simulink model "solucion"  (R2021a)
settings: Solver=VariableStepAuto  StartTime=0.0  StopTime=1435  RelTol=1e-3
values from neighbouring files (symbols this model uses):
  radiacion_solar = flip(radiacion_solar)    [setup.m]
  temperatura = flip(temperatura)    [setup.m]
  tiempo = 1:5:1436    [setup.m]
  tiempo_temperatura = tiempo(indices)    [setup.m]
libraries: spsCurrentMeasurementLib x1, spsPVArrayLib x1, spsSeriesRLCBranchLib x1, spsVoltageMeasurementLib x1, spspowerguiLib x1
settings Model: Creator=MarcosRPesanteColón  LastModifiedBy=MarcosRPesanteColón

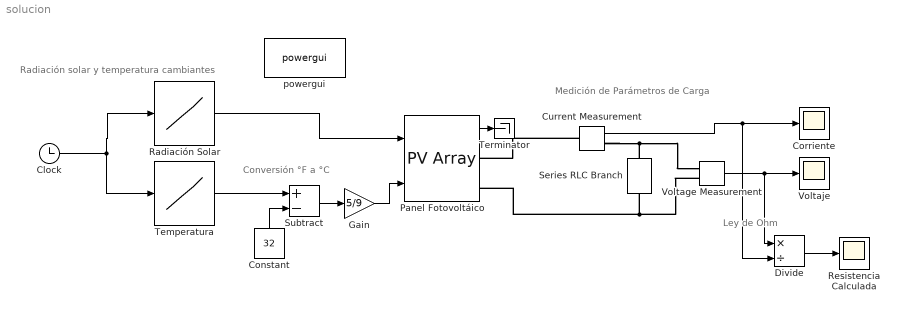
== system solucion ==
  note: Medición de Parámetros de Carga
  note: Radiación solar y
      | temperatura
      | cambiantes
  note: Ley de Ohm
  note: Conversión °F a °C
  Clock : Clock
  Constant : Constant  Value=32
  Corriente : Scope
  Current Measurement : spsCurrentMeasurementLib/Current Measurement  PhasorSimulation=off  OutputType=Complex  PSBequivalent=0
  Divide : Product  Inputs=*/
  Gain : Gain  Gain=5/9
  Panel Fotovoltáico : spsPVArrayLib/PV Array  Npar=1  Nser=1  PlotType=array @ 1000 W/m2 & specified temperatures  S_vec="[ 1000  500  100 ]"  Temp_C_vec="[ 45 25  ]"  ModuleName=REC Solar REC280TP BLK2  PlotWhenSelected=off  Pm=280.158  Ncell=60  Voc=38.7  Isc=9.46  Vm=31.8  Im=8.81  beta_Voc_pc=-0.31  alpha_Isc_pc=0.05  beta_Voc=-0.11997  alpha_Isc=0.00473  IL=9.4771  I0=4.8375e-11  nI=0.96658  Rsh=147.5721  Rs=0.26708  RobustModel=off  RobustCellTemperature=313.3991  BAL=on  Tc=1e-6  Tfilter=5e-5
  Radiación Solar : Lookup_n-D  NumberOfTableDimensions=1  BreakpointsForDimension1=tiempo  Table=radiacion_solar  InternalRulePriority=Speed  RndMeth=Simplest  InputSameDT=on
  Resistencia Calculada : Scope
  Series RLC Branch : spsSeriesRLCBranchLib/Series RLC Branch  LConnTagsString=__new0  RConnTagsString=__new0  BranchType=R  Resistance=5  Inductance=0  SetiL0=off  InitialCurrent=0  Capacitance=0  Setx0=off  InitialVoltage=0  Measurements=None
  Subtract : Sum  Inputs=+-
  Temperatura : Lookup_n-D  NumberOfTableDimensions=1  BreakpointsForDimension1=tiempo_temperatura  Table=temperatura  InternalRulePriority=Speed  RndMeth=Simplest  InputSameDT=on
  Terminator : Terminator
  Voltage Measurement : spsVoltageMeasurementLib/Voltage Measurement  PhasorSimulation=off  OutputType=Complex  PSBequivalent=0
  Voltaje : Scope
  powergui : spspowerguiLib/powergui  Priority=1  SimulationMode=Continuous  SampleTime=50e-6  frequency=60  Iterations=50  frequencyindice=0  Pbase=100e6  ErrMax=1e-4  UnitsV=kV  UnitsW=MW  buscounter=0  FunctionMessages=off  echomessages=off  EnableUseOfTLC=off  CurrentSourceSwitches=off  DisableSnubberDevices=off  DisableRonSwitches=off  DisableVfSwitches=off  DisplayEquations=off  AutomaticDiscreteSolvers=off  SolverType=Tustin/Backward Euler (TBE)  Interpol=off  ExternalGateDelay=off  methode=off  Ts=100  x0status=blocks  SPID=on  SwTol=0  HookPort=off  NonlinearTolerance=1e-4  nMaxIteration=100  ContinueOnMaxIteration=off  RestoreLinks=warning  ResistiveCurrentMeasurement=off  Frange=[0:2:500]  Ylog=off  Xlog=on  ShowGrid=off  save=off  variable=ZData  structure=0  ZoomFFT=off  StartTime=0.0  cycles=1  DisplayStyle=1  fundamental=60  FreqAxis=off  MaxFrequency=1000  frequencyindicesteady=1  RmsSteady=1  display=off
  wires:
  Radiación Solar/1 -> Panel Fotovoltáico/1
  Clock/1 -> Radiación Solar/1, Temperatura/1
  Voltage Measurement/1 -> Divide/1, Voltaje/1
  Current Measurement/1 -> Corriente/1, Divide/2
  Constant/1 -> Subtract/2
  Temperatura/1 -> Subtract/1
  Subtract/1 -> Gain/1
  Gain/1 -> Panel Fotovoltáico/2
  Divide/1 -> Resistencia Calculada/1
  Panel Fotovoltáico/1 -> Terminator/1
  connections:
  Current Measurement/RConn1 -- Voltage Measurement/LConn1 -- Series RLC Branch/LConn1
  Voltage Measurement/LConn2 -- Series RLC Branch/RConn1 -- Panel Fotovoltáico/RConn2
  Current Measurement/LConn1 -- Panel Fotovoltáico/RConn1
